simulink model "QuadRotor_Simulink_Aksland"  (R2021b)
settings: Solver=ode23tb  StartTime=0.0  StopTime=50  RelTol=1e-3
values from neighbouring files (symbols this model uses):
  A = qrs.LinearPlantModel.A    [ControllerDev.m]    (also in ControllerDev_Aksland.m)
  B = qrs.LinearPlantModel.B    [ControllerDev.m]    (also in ControllerDev_Aksland.m)
  C = eye(size(A))    [ControllerDev.m]    (also in ControllerDev_Aksland.m = qrs.LinearPlantModel.C)
  D = zeros(size(C,1),size(B,2))    [ControllerDev.m]    (also in ControllerDev_Aksland.m)
  K = zeros(size(B,2), size(A,1), numel(t))    [ControllerDev.m]    (also in ControllerDev_Aksland.m = lqr(A,B,Q,R))
  K_tilde = -inv(C*inv(A-B*K)*B)    [ControllerDev_Aksland.m]
undefined symbols (not defined in the file or in its folder): QR_Object
libraries: uavutilslib x1
settings Model: Creator=renkert2  LastModifiedBy=renkert2
settings SolverCC: AlgebraicLoopSolver=TrustRegion
settings DebuggingCC: SFMachineParentedDataDiag=warning

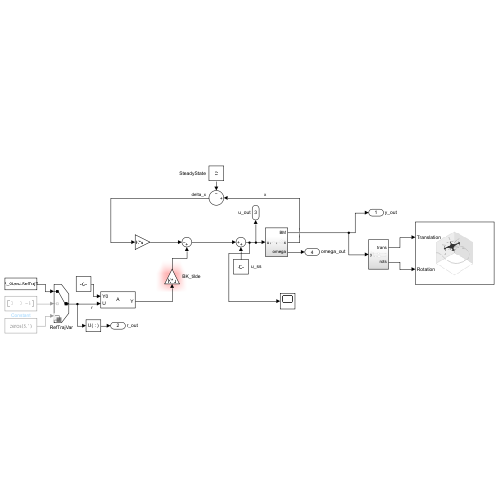
[thumbnail: Simulink's stored preview of the top-level diagram]
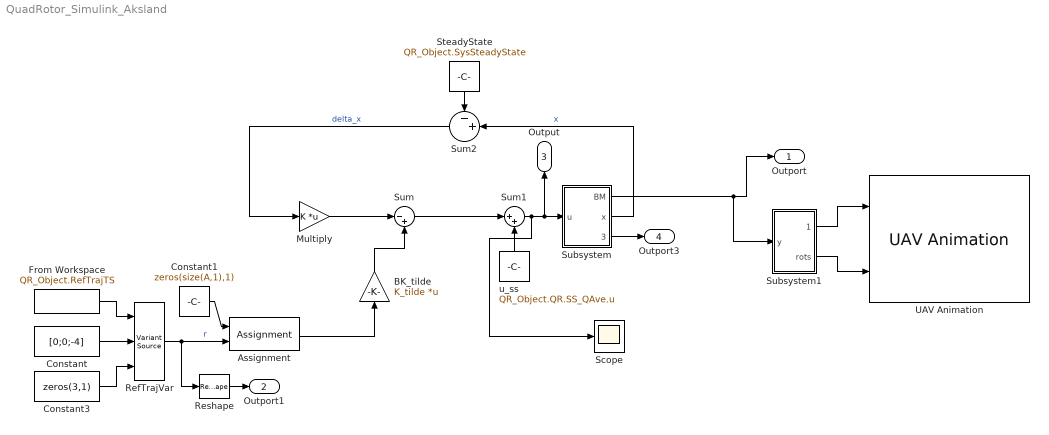
== system QuadRotor_Simulink_Aksland ==
  Assignment : Assignment  DiagnosticForDimensions=Warning  IndexOptions=Index vector (dialog)  Indices=[5 6 7]  OutputSizes=1
  BK_tilde : Gain  Gain=K_tilde  Multiplication=Matrix(K*u)
  Constant : Constant  Value=[0;0;-4]
  Constant1 : Constant  Value=zeros(size(A,1),1)
  Constant3 : Constant  Value=zeros(3,1)
  From Workspace : FromWorkspace  VariableName=QR_Object.RefTrajTS  OutputAfterFinalValue=Holding final value
  Multiply : Gain  Gain=K  Multiplication=Matrix(K*u)
  RefTrajVar : VariantSource  VariantControlMode=label  LabelModeActiveChoice=TimeSeries
  Reshape : Reshape
  Scope : Scope
  SteadyState : Constant  Value=QR_Object.SysSteadyState
  Subsystem : Subsystem
  Subsystem1 : Subsystem
  Sum : Sum  Inputs=|-+
  Sum1 : Sum  Inputs=|++
  Sum2 : Sum  Inputs=-+|
  UAV Animation : uavutilslib/UAV Animation  UAVType=Multirotor  UAVSize=1  InertialZDirection=Down  SampleTime=-1
      settings: SourceProductBaseCode=UV
  u_ss : Constant  Value=QR_Object.QR.SS_QAve.u  VectorParams1D=off
  Outport : Outport  SignalName=y_out
  Outport1 : Outport  Port=2  SignalName=r_out
  Output : Outport  Port=3  SignalName=u_out
  Outport3 : Outport  Port=4  SignalName=omega_out
  wires:
  From Workspace/1 -> RefTrajVar/1
  Reshape/1 -> Outport1/1
  Subsystem/1(BM) -> Subsystem1/1(y), Outport/1
  Constant/1 -> RefTrajVar/2
  RefTrajVar/1 -> Assignment/2, Reshape/1  "r"
  Subsystem/2(x) -> Sum2/2  "x"
  u_ss/1 -> Sum1/2
  Sum1/1 -> Scope/1, Subsystem/1(u), Output/1
  Subsystem/3(omega) -> Outport3/1
  Multiply/1 -> Sum/1
  Constant3/1 -> RefTrajVar/3
  SteadyState/1 -> Sum2/1
  Sum2/1 -> Multiply/1  "delta_x"
  Sum/1 -> Sum1/1
  Constant1/1 -> Assignment/1
  Assignment/1 -> BK_tilde/1
  BK_tilde/1 -> Sum/2
  Subsystem1/1(trans) -> UAV Animation/1
  Subsystem1/2(rots) -> UAV Animation/2

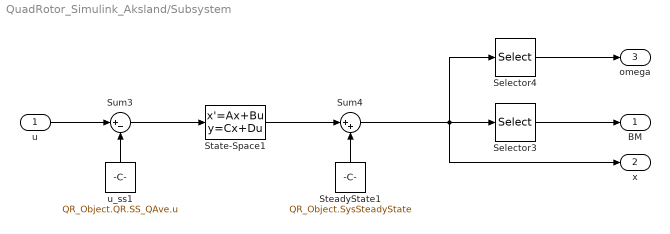
== system QuadRotor_Simulink_Aksland/Subsystem ==
  u : Inport
  Selector3 : Selector  InputPortWidth=16  IndexOptions=Index vector (dialog)  Indices=5:16  OutputSizes=1
  Selector4 : Selector  InputPortWidth=16  IndexOptions=Index vector (dialog)  Indices=1:4  OutputSizes=1
  State-Space1 : StateSpace  A=A  B=B  C=C  D=D  InitialCondition=0
  SteadyState1 : Constant  Value=QR_Object.SysSteadyState
  Sum3 : Sum  Inputs=|+-
  Sum4 : Sum  Inputs=|++
  u_ss1 : Constant  Value=QR_Object.QR.SS_QAve.u  VectorParams1D=off
  BM : Outport
  x : Outport  Port=2
  omega : Outport  Port=3
  wires:
  Sum4/1 -> x/1, Selector4/1, Selector3/1
  u_ss1/1 -> Sum3/2
  State-Space1/1 -> Sum4/1
  SteadyState1/1 -> Sum4/2
  u/1 -> Sum3/1
  Selector3/1 -> BM/1
  Selector4/1 -> omega/1
  Sum3/1 -> State-Space1/1

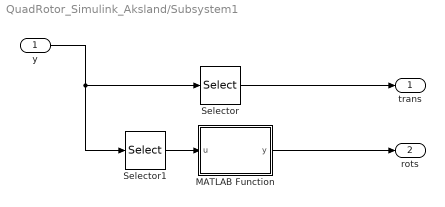
== system QuadRotor_Simulink_Aksland/Subsystem1 ==
  y : Inport
  MATLAB Function : MATLAB Function  TreatAsAtomicUnit=on
  Selector : Selector  InputPortWidth=QR_Object.QR.BM.Nx  IndexOptions=Index vector (dialog)  Indices=QR_Object.QR.BM.I.x.p  OutputSizes=1
  Selector1 : Selector  InputPortWidth=QR_Object.QR.BM.Nx  IndexOptions=Index vector (dialog)  Indices=QR_Object.QR.BM.I.x.Theta  OutputSizes=1
  trans : Outport
  rots : Outport  Port=2
  wires:
  Selector/1 -> trans/1
  Selector1/1 -> MATLAB Function/1(u)
  y/1 -> Selector/1, Selector1/1
  MATLAB Function/1(y) -> rots/1

== matlab function QuadRotor_Simulink_Aksland/Subsystem1/MATLAB Function ==
  data: u input; y output
function y = eul2quatMF(u)
    y = eul2quat([1 -1 1].*fliplr(u'),'ZYX');
end
